simulink model "controle_pid_div_acao"  (R2018b)
settings: Solver=VariableStepAuto  StartTime=0.0  StopTime=1000  RelTol=1e-3
values from neighbouring files (symbols this model uses):
  b = 0    [simula_div_acao_pond.m]    (also in simula_div_acao_pond2.m = 0.5; simula_div_acao_trad.m = 1)
  c = 0    [simula_div_acao_pond.m]    (also in simula_div_acao_pond2.m = 0.5; simula_div_acao_trad.m = 1)
  h10 = 25    [dadosTanque.m]
  h20 = 20    [dadosTanque.m]
  k1 = 25    [dadosTanque.m]
  k2 = 25    [dadosTanque.m]
  kac = 20    [dadosTanque.m]
  q10 = k1*sqrt(h10) + kac*sqrt(h10-h20)    [dadosTanque.m]
  q20 = k2*sqrt(h20) - kac*sqrt(h10-h20)    [dadosTanque.m]
  sw_noise = 0    [simula_anti_windup.m]    (also in simula_d_filter.m = 1; simula_div_acao_pond.m = 1; simula_div_acao_pond2.m = 1; simula_div_acao_trad.m = 1)
  ts = 0.01    [Atividade3.m]
undefined symbols (not defined in the file or in its folder): pid_var
settings Model: Creator=Caléo  LastModifiedBy=Caléo

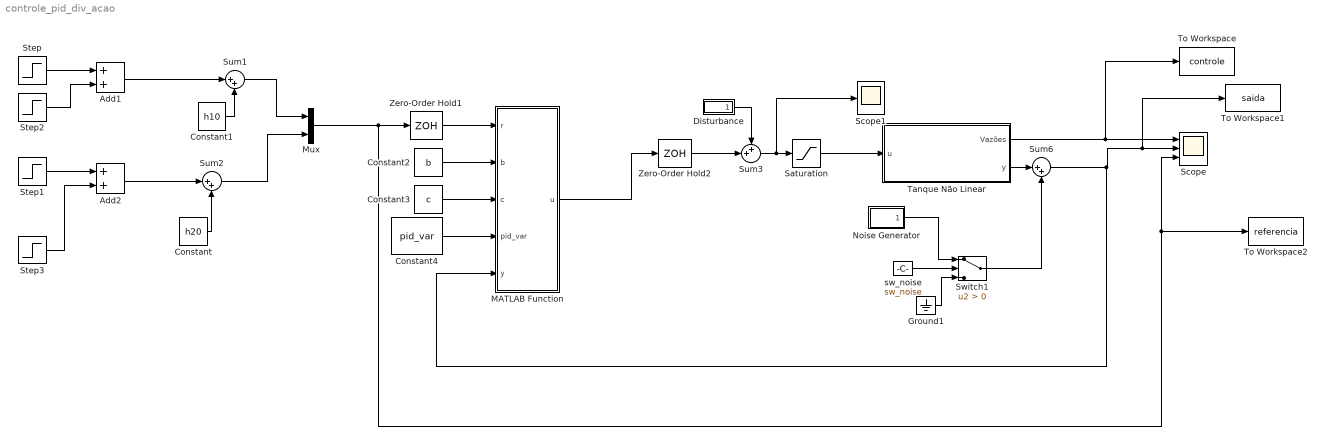
== system controle_pid_div_acao ==
  Add1 : Sum
  Add2 : Sum
  Constant : Constant  Value=h20
  Constant1 : Constant  Value=h10
  Constant2 : Constant  Value=b
  Constant3 : Constant  Value=c
  Constant4 : Constant  Value=pid_var  OutDataTypeStr=Bus: pid_var_bus
  Disturbance : Subsystem
  Ground1 : Ground
  MATLAB Function : MATLAB Function  TreatAsAtomicUnit=on
  Mux : Mux  Inputs=2
  Noise Generator : Subsystem
  Saturation : Saturate  UpperLimit=[0.2*q10 0.2*q20]  LowerLimit=[-q10 ;-q20]
  Scope : Scope  NumInputPorts=3
  Scope1 : Scope
  Step : Step  After=5  SampleTime=0
  Step1 : Step  After=3  SampleTime=0
  Step2 : Step  Time=300  After=-6  SampleTime=0
  Step3 : Step  Time=300  After=-6  SampleTime=0
  Sum1 : Sum  Inputs=|++
  Sum2 : Sum  Inputs=|++
  Sum3 : Sum  Inputs=++|
  Sum6 : Sum  Inputs=|++
  Switch1 : Switch  Criteria=u2 > Threshold
  Tanque Não Linear : Subsystem
  To Workspace : ToWorkspace  VariableName=controle  SaveFormat=Timeseries  SampleTime=-1
  To Workspace1 : ToWorkspace  VariableName=saida  SaveFormat=Timeseries  SampleTime=-1
  To Workspace2 : ToWorkspace  VariableName=referencia  SaveFormat=Timeseries  SampleTime=-1
  Zero-Order Hold1 : ZeroOrderHold  SampleTime=ts
  Zero-Order Hold2 : ZeroOrderHold  SampleTime=ts
  sw_noise : Constant  Value=sw_noise
  wires:
  Tanque Não Linear/1(Vazões) -> To Workspace/1, Scope/1
  Step3/1 -> Add2/2
  Sum1/1 -> Mux/1
  Constant1/1 -> Sum1/2
  Sum2/1 -> Mux/2
  Sum6/1 -> MATLAB Function/5(y), To Workspace1/1, Scope/2
  Tanque Não Linear/2(y) -> Sum6/1
  Add2/1 -> Sum2/1
  Step1/1 -> Add2/1
  Step2/1 -> Add1/2
  Noise Generator/1(Out1) -> Switch1/1
  Saturation/1 -> Tanque Não Linear/1(u)
  Ground1/1 -> Switch1/3
  sw_noise/1 -> Switch1/2
  Step/1 -> Add1/1
  Add1/1 -> Sum1/1
  Switch1/1 -> Sum6/2
  Constant/1 -> Sum2/2
  Constant2/1 -> MATLAB Function/2(b)
  Constant3/1 -> MATLAB Function/3(c)
  Constant4/1 -> MATLAB Function/4(pid_var)
  Mux/1 -> Zero-Order Hold1/1, To Workspace2/1, Scope/3
  Zero-Order Hold1/1 -> MATLAB Function/1(r)
  MATLAB Function/1(u) -> Zero-Order Hold2/1
  Disturbance/1(Out1) -> Sum3/1
  Zero-Order Hold2/1 -> Sum3/2
  Sum3/1 -> Scope1/1, Saturation/1

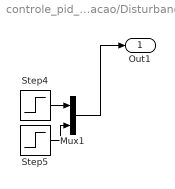
== system controle_pid_div_acao/Disturbance ==
  Mux1 : Mux  Inputs=2
  Step4 : Step  Time=600  After=10  SampleTime=0
  Step5 : Step  Time=600  After=10  SampleTime=0
  Out1 : Outport
  wires:
  Step5/1 -> Mux1/2
  Mux1/1 -> Out1/1
  Step4/1 -> Mux1/1

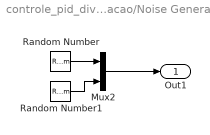
== system controle_pid_div_acao/Noise Generator ==
  Mux2 : Mux  Inputs=2
  Random Number : RandomNumber  Variance=0.01  SampleTime=0.1
  Random Number1 : RandomNumber  Variance=0.01  SampleTime=0.1
  Out1 : Outport
  wires:
  Random Number1/1 -> Mux2/2
  Random Number/1 -> Mux2/1
  Mux2/1 -> Out1/1

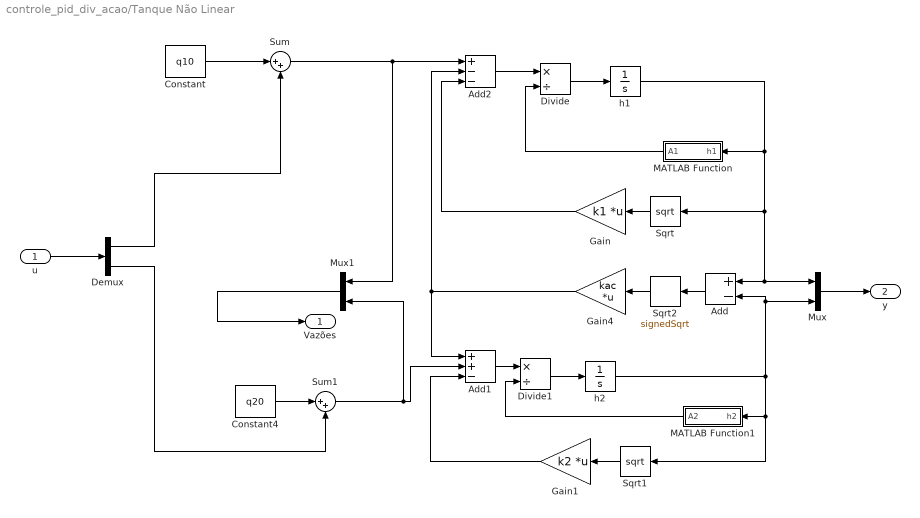
== system controle_pid_div_acao/Tanque Não Linear ==
  u : Inport
  Add : Sum  Inputs=+-
  Add1 : Sum  Inputs=++-
  Add2 : Sum  Inputs=+--
  Constant : Constant  Value=q10
  Constant4 : Constant  Value=q20
  Demux : Demux  Outputs=2
  Divide : Product  Inputs=*/
  Divide1 : Product  Inputs=*/
  Gain : Gain  Gain=k1  Multiplication=Matrix(K*u)
  Gain1 : Gain  Gain=k2  Multiplication=Matrix(K*u)
  Gain4 : Gain  Gain=kac  Multiplication=Matrix(K*u)
  MATLAB Function : MATLAB Function  TreatAsAtomicUnit=on
  MATLAB Function1 : MATLAB Function  TreatAsAtomicUnit=on
  Mux : Mux  Inputs=2
  Mux1 : Mux  Inputs=2
  Sqrt : Sqrt  SaturateOnIntegerOverflow=on
  Sqrt1 : Sqrt  SaturateOnIntegerOverflow=on
  Sqrt2 : Sqrt  Operator=signedSqrt  SaturateOnIntegerOverflow=on
  Sum : Sum  Inputs=|++
  Sum1 : Sum  Inputs=|++
  h1 : Integrator  InitialCondition=h10  LimitOutput=on  UpperSaturationLimit=50  LowerSaturationLimit=0
  h2 : Integrator  InitialCondition=h20  LimitOutput=on  UpperSaturationLimit=50  LowerSaturationLimit=0
  Vazões : Outport
  y : Outport  Port=2
  wires:
  u/1 -> Demux/1
  h2/1 -> Add/2, Mux/2, MATLAB Function1/1(h2), Sqrt1/1
  Sqrt2/1 -> Gain4/1
  Gain/1 -> Add2/3
  Demux/1 -> Sum/2
  Demux/2 -> Sum1/2
  Divide/1 -> h1/1
  h1/1 -> Mux/1, Add/1, Sqrt/1, MATLAB Function/1(h1)
  Add/1 -> Sqrt2/1
  Mux1/1 -> Vazões/1
  Gain4/1 -> Add2/2, Add1/1
  Sqrt1/1 -> Gain1/1
  Constant/1 -> Sum/1
  Divide1/1 -> h2/1
  Constant4/1 -> Sum1/1
  Add1/1 -> Divide1/1
  MATLAB Function1/1(A2) -> Divide1/2
  Add2/1 -> Divide/1
  MATLAB Function/1(A1) -> Divide/2
  Gain1/1 -> Add1/3
  Mux/1 -> y/1
  Sqrt/1 -> Gain/1
  Sum/1 -> Mux1/1, Add2/1
  Sum1/1 -> Mux1/2, Add1/2

== matlab function controle_pid_div_acao/Tanque Não Linear/MATLAB Function1 ==
  data: h2 input; A2 output
function A2 = secao_tanque(h2)

    if h2 < 7.5
        d2 = 6; 
    elseif h2 < 19.5
        d2 = (19.5 - h2)/2;
    elseif h2 < 29.5
        d2 = 0;
    elseif h2 < 41.5
        d2=(h2 - 29.5)/2;
    elseif h2 >= 41.5
        d2 = 6;
    else 
        d2 = 6;
    end
    A2 = 9*(14+d2);
    
end

== matlab function controle_pid_div_acao/Tanque Não Linear/MATLAB Function ==
  data: h1 input; A1 output
function A1 = secao_tanque(h1)

    if h1 < 7.5
        d1 = 0;
    elseif h1 < 19.5
        d1 = (h1 - 7.5)/2;
    elseif h1 < 29.5
        d1 = 6;
    elseif h1 < 41.5
        d1 = (41.5 - h1)/2;
    elseif h1 >= 41.5
        d1 = 0;
    else 
        d1 = 0;
    end
    A1 = 9*(8+d1);
end

== matlab function controle_pid_div_acao/MATLAB Function ==
  settings: updateMethod=DISCRETE
  data: r input; b input; c input; pid_var input; y input; u output
function u = pid_div_acao(r,b,c,pid_var,y)
persistent e_d_p e_acum_p acao_d_p

Kp = pid_var.Kp;
Ki = pid_var.Ki ;
Td = pid_var.Td;


Kp = Kp*[1 1]';

Ki = Ki*[1 1]';

Td = Td*[1 1]';




[m,n] = size(Kp);
    if isempty(e_d_p)
        e_d_p = zeros(m,1);
    end
    
    if isempty(e_acum_p)
        e_acum_p = zeros(m,1);
    end
    
    if isempty(acao_d_p)
        acao_d_p = zeros(m,1);
    end
        

u = zeros(m,1);


Tf = 100;
ts = 0.01;
a = ts/(Tf+ts);

for i=1:m
    e_acum = (r(i)-y(i)) + e_acum_p(i);
    acao_p = b*r(i)-y(i);
    acao_i = Ki(i)*e_acum*ts;
    acao_d = Td(i)*((c*r(i)-y(i))-e_d_p(i))/ts;
    acao_d_filt = (1-a)*acao_d_p(i) + a*(acao_d);
    
    u(i) = Kp(i)*(acao_p + acao_i + acao_d_filt);
    
    acao_d_p(i) = acao_d_filt;
    e_acum_p(i) = e_acum;
    e_d_p(i) = c*r(i)-y(i);

    
end






end
